simulink model "sfcndemo_sfun_rtwdwork"  (Simulink 6.0)
settings: Solver=FixedStepDiscrete  StartTime=0.0  StopTime=10.0  FixedStep=1  RelTol=1e-3
settings Model: Creator=The MathWorks Inc.  LastModifiedBy=batserve  ExtModeAutoUpdateStatusClock=off
settings OptimizationCC: BooleanDataType=off  InlineParams=on  InlineInvariantSignals=off  ZeroExternalMemoryAtStartup=off  ZeroInternalMemoryAtStartup=off  OptimizeModelRefInitCode=on  LifeSpan=1
settings DebuggingCC: CheckExecutionContextPreStartOutputMsg=on  CheckExecutionContextRuntimeOutputMsg=on  SolverPrmCheckMsg=none
settings HardwareCC: TargetUnknown=on
settings RTWCC: SystemTargetFile=ert.tlc  GenCodeOnly=on  TemplateMakefile=ert_default_tmf  ProcessScript=ert_make_rtw_hook
settings CodeAppCC: IgnoreCustomStorageClasses=off
settings ERTTargetCC: TargetFcnLib=ansi_tfl_tmw.mat  GenFloatMathFcnCalls=ANSI_C  GenerateSampleERTMain=on  SupportContinuousTime=on  SupportNonInlinedSFcns=on  InlinedParameterPlacement=NonHierarchical  RootIOFormat=Individual Arguments  ERTCustomFileTemplate=example_file_process.tlc  InitialValueSource=Model

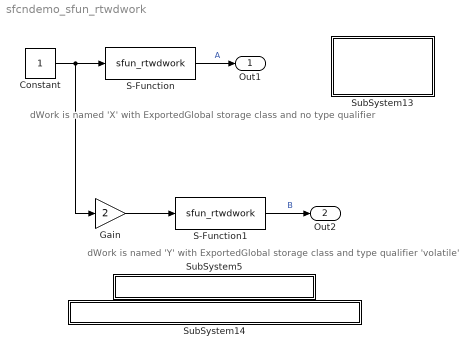
== system sfcndemo_sfun_rtwdwork ==
  note: dWork is named 'X' with ExportedGlobal
      | storage class and no type qualifier
  note: dWork is named 'Y' with ExportedGlobal
      | storage class and type qualifier 'volatile'
  Constant : Constant
  Gain : Gain  Gain=2
  S-Function : S-Function  FunctionName=sfun_rtwdwork  Parameters=id,sc,tq  mask{id='X', sc=ExportedGlobal, tq=''}
      mask prompts: id "RTW Identifier"; sc "RTW Storage Class"; tq "RTW Type Qualifier"
      mask StyleString: edit,popup(Auto|ExportedGlobal|ImportedExtern|ImportedExternPointer),edit
  S-Function1 : S-Function  FunctionName=sfun_rtwdwork  Parameters=id,sc,tq  mask{id='Y', sc=ExportedGlobal, tq='volatile'}
      mask prompts: id "RTW Identifier"; sc "RTW Storage Class"; tq "RTW Type Qualifier"
      mask StyleString: edit,popup(Auto|ExportedGlobal|ImportedExtern|ImportedExternPointer),edit
  SubSystem13 : Subsystem  PropExecContextAcrossSSBoundary=on
      settings: OpenFcn=rtwdwork_inspect('sfcndemo_sfun_rtwdwork.c');
      mask Display: disp('Generate and\ninspect code')
  SubSystem14 : Subsystem  PropExecContextAcrossSSBoundary=on  mask{filename=sfun_rtwdwork.tlc}
      mask prompts: filename "file name"
      mask init:
      | x=sfundemo_maskdisp;
      settings: AttributesFormatString=\n\n\n\n\n\n\n\n\n\n  OpenFcn=sfundemo_openfcn
      mask Display: disp(x)
  SubSystem5 : Subsystem  PropExecContextAcrossSSBoundary=on  mask{filename=sfun_rtwdwork.c}
      mask prompts: filename "file name"
      mask init:
      | x=sfundemo_maskdisp;
      settings: AttributesFormatString=\n\n\n\n\n\n\n\n\n\n  OpenFcn=sfundemo_openfcn
      mask Display: disp(x)
  Out1 : Outport
  Out2 : Outport  Port=2
  wires:
  Constant/1 -> S-Function/1, Gain/1
  S-Function/1 -> Out1/1  "A"
  S-Function1/1 -> Out2/1  "B"
  Gain/1 -> S-Function1/1

== system sfcndemo_sfun_rtwdwork/SubSystem13 ==

== system sfcndemo_sfun_rtwdwork/SubSystem14 ==

== system sfcndemo_sfun_rtwdwork/SubSystem5 ==
